simulink model "Sample594"  (R2021b)
settings: Solver=VariableStepAuto  StartTime=0.0  StopTime=10.0  RelTol=1e-3
undefined symbols (not defined in the file): DiscIntNeverNeededParam, magnitude, Newton, Raphson
libraries: simulink x402, pid_lib x98
(part 1 of 14)
settings Model: Creator=user  LastModifiedBy=汪海博

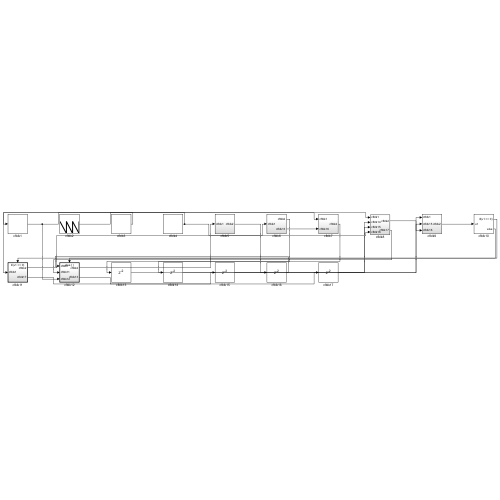
[thumbnail: Simulink's stored preview of the top-level diagram]
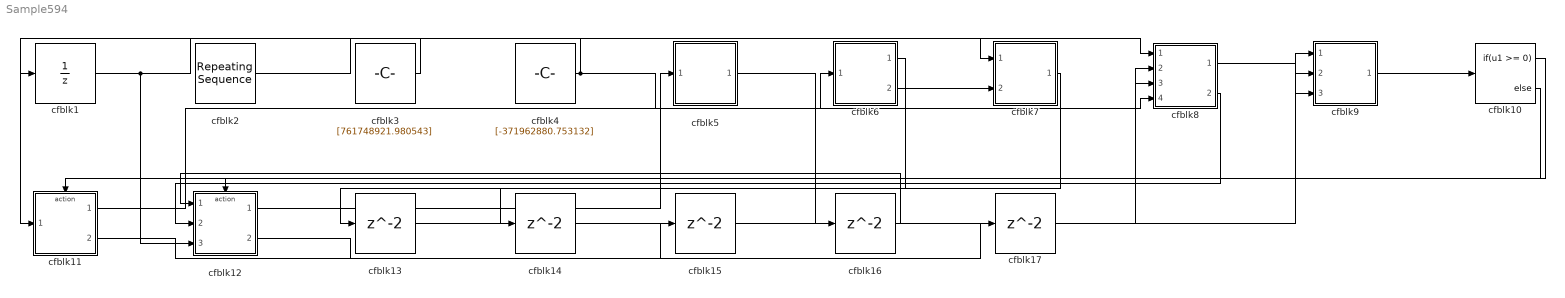
== system Sample594 ==
  cfblk1 : UnitDelay  HasFrameUpgradeWarning=on
  cfblk10 : If  IfExpression=u1 >= 0  SampleTime=1
  cfblk11 : Subsystem  TreatAsAtomicUnit=on
  cfblk12 : Subsystem  TreatAsAtomicUnit=on
  cfblk{13..17} (5 alike) : Delay  SampleTime=1
  cfblk2 : simulink/Sources/Repeating Sequence  rep_seq_t=[0 2]  rep_seq_y=[-284129757.481176, -754756546.872150]
  cfblk3 : Constant  Value=[761748921.980543]  SampleTime=1
  cfblk4 : Constant  Value=[-371962880.753132]  SampleTime=1
  cfblk5 : Subsystem
  cfblk6 : Subsystem
  cfblk7 : Subsystem
  cfblk8 : Subsystem
  cfblk9 : Subsystem
  wires:
  cfblk11/1(cfblk2) -> cfblk6/1(cfblk1)
  cfblk4/1 -> cfblk11/1(cfblk1), cfblk8/4(cfblk16)
  cfblk2/1 -> cfblk7/1(cfblk1)
  cfblk9/1(cfblk2) -> cfblk10/1
  cfblk3/1 -> cfblk1/1
  cfblk1/1 -> cfblk8/1(cfblk1), cfblk12/3(cfblk12)
  cfblk8/1(cfblk2) -> cfblk9/3(cfblk16)
  cfblk12/1(cfblk2) -> cfblk5/1(cfblk1)
  cfblk6/2(cfblk13) -> cfblk7/2(cfblk16)
  cfblk8/2(cfblk17) -> cfblk12/2(cfblk11)
  cfblk10/1 -> cfblk11/Action
  cfblk10/2 -> cfblk12/Action
  cfblk6/1(cfblk2) -> cfblk13/1
  cfblk13/1 -> cfblk9/2(cfblk15)
  cfblk7/1(cfblk2) -> cfblk14/1
  cfblk14/1 -> cfblk8/2(cfblk14)
  cfblk11/2(cfblk17) -> cfblk15/1
  cfblk15/1 -> cfblk9/1(cfblk1)
  cfblk5/1(cfblk2) -> cfblk16/1
  cfblk16/1 -> cfblk12/1(cfblk1)
  cfblk12/2(cfblk13) -> cfblk17/1
  cfblk17/1 -> cfblk8/3(cfblk15)

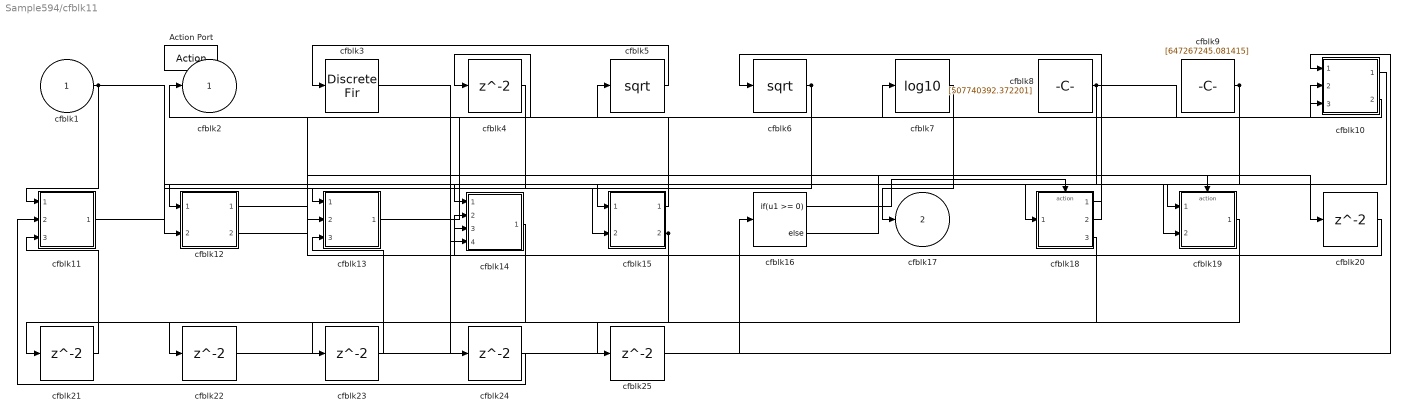
== system Sample594/cfblk11 ==
  cfblk1 : Inport
  Action Port : ActionPort  ActionPortLabel=if(u1 >= 0)
  cfblk10 : Subsystem
  cfblk11 : Subsystem
  cfblk12 : Subsystem
  cfblk13 : Subsystem
  cfblk14 : Subsystem
  cfblk15 : Subsystem
  cfblk16 : If  IfExpression=u1 >= 0  SampleTime=1
  cfblk18 : Subsystem  TreatAsAtomicUnit=on
  cfblk19 : Subsystem  TreatAsAtomicUnit=on
  cfblk{4,20..25} (7 alike) : Delay
  cfblk3 : DiscreteFir
  cfblk5 : Sqrt  SaturateOnIntegerOverflow=on
  cfblk6 : Sqrt  SaturateOnIntegerOverflow=on
  cfblk7 : Math  Operator=log10  SaturateOnIntegerOverflow=on
  cfblk8 : Constant  Value=[507740392.372201]  SampleTime=1
  cfblk9 : Constant  Value=[647267245.081415]  SampleTime=1
  cfblk2 : Outport
  cfblk17 : Outport  Port=2
  wires:
  cfblk1/1 -> cfblk11/1(cfblk1), cfblk19/2(cfblk8), cfblk15/2(cfblk9)
  cfblk8/1 -> cfblk12/1(cfblk1), cfblk10/3(cfblk15)
  cfblk11/1(cfblk2) -> cfblk13/1(cfblk1)
  cfblk18/1(cfblk2) -> cfblk6/1
  cfblk4/1 -> cfblk12/2(cfblk14)
  cfblk6/1 -> cfblk4/1, cfblk14/4(cfblk15)
  cfblk9/1 -> cfblk19/1(cfblk1), cfblk14/1(cfblk1)
  cfblk5/1 -> cfblk3/1
  cfblk12/2(cfblk15) -> cfblk7/1
  cfblk7/1 -> cfblk17/1
  cfblk18/2(cfblk12) -> cfblk15/1(cfblk1)
  cfblk15/1(cfblk2) -> cfblk2/1
  cfblk10/1(cfblk2) -> cfblk18/1(cfblk1)
  cfblk15/2(cfblk10) -> cfblk14/2(cfblk13), cfblk14/3(cfblk14), cfblk22/1
  cfblk13/1(cfblk2) -> cfblk10/2(cfblk14)
  cfblk10/2(cfblk16) -> cfblk5/1
  cfblk16/1 -> cfblk18/Action
  cfblk16/2 -> cfblk19/Action
  cfblk12/1(cfblk2) -> cfblk20/1
  cfblk20/1 -> cfblk13/2(cfblk10)
  cfblk14/1(cfblk2) -> cfblk21/1
  cfblk21/1 -> cfblk11/3(cfblk15)
  cfblk22/1 -> cfblk10/1(cfblk1)
  cfblk18/3(cfblk13) -> cfblk23/1
  cfblk23/1 -> cfblk13/3(cfblk11)
  cfblk3/1 -> cfblk24/1
  cfblk24/1 -> cfblk11/2(cfblk14)
  cfblk19/1(cfblk2) -> cfblk25/1
  cfblk25/1 -> cfblk16/1

== system Sample594/cfblk12 ==
  cfblk1 : Inport
  cfblk11 : Inport  Port=2
  cfblk12 : Inport  Port=3
  Action Port : ActionPort  ActionPortLabel=else
  cfblk10 : Subsystem
  cfblk14 : Delay
  cfblk3 : simulink/Discrete/Transfer Fcn Lead or Lag  PoleZ=0.95  ZeroZ=0.75  ICPrevOutput=0.0  ICPrevInput=0.0  DoSatur=off
      settings: SourceProductBaseCode=SL
  cfblk4 : Product  Inputs=*
  cfblk5 : Product  Inputs=**
  cfblk6 : Abs
  cfblk7 : Sum  Inputs=+-
  cfblk8 : Constant  Value=[-306003779.164927]  SampleTime=1
  cfblk9 : Subsystem
  cfblk2 : Outport
  cfblk13 : Outport  Port=2
  wires:
  cfblk6/1 -> cfblk9/1(cfblk1)
  cfblk11/1 -> cfblk7/1
  cfblk3/1 -> cfblk7/2, cfblk10/2(cfblk11)
  cfblk1/1 -> cfblk5/1
  cfblk8/1 -> cfblk4/1
  cfblk4/1 -> cfblk3/1
  cfblk10/1(cfblk2) -> cfblk13/1
  cfblk12/1 -> cfblk2/1
  cfblk7/1 -> cfblk5/2
  cfblk5/1 -> cfblk10/1(cfblk1)
  cfblk9/1(cfblk2) -> cfblk14/1
  cfblk14/1 -> cfblk6/1

== system Sample594/cfblk5 ==
  cfblk1 : Inport
  cfblk3 : simulink/Math Operations/MinMax Running Resettable  Function=min  vinit=0.0
  cfblk4 : Gain  Gain=[768236273.683915]
  cfblk5 : ComplexToMagnitudeAngle
  cfblk6 : Product  Inputs=**
  cfblk7 : Constant  Value=[-650989527.079987]  SampleTime=1
  cfblk8 : Subsystem
  cfblk9 : Delay  SampleTime=1
  cfblk2 : Outport
  wires:
  cfblk3/1 -> cfblk8/1(cfblk1)
  cfblk4/1 -> cfblk6/1
  cfblk7/1 -> cfblk8/2(cfblk9)
  cfblk8/1(cfblk2) -> cfblk4/1
  cfblk8/2(cfblk10) -> cfblk2/1
  cfblk1/1 -> cfblk5/1
  cfblk5/1 -> cfblk3/2
  cfblk5/2 -> cfblk6/2
  cfblk6/1 -> cfblk9/1
  cfblk9/1 -> cfblk3/1

== system Sample594/cfblk6 ==
  cfblk1 : Inport
  cfblk10 : Subsystem
  cfblk11 : Subsystem
  cfblk12 : Subsystem
  cfblk{3,14..18} (6 alike) : Delay  SampleTime=1
  cfblk4 : DiscreteFir  SampleTime=1
  cfblk5 : DotProduct  InputSameDT=on  OutDataTypeStr=Inherit: Inherit via internal rule
  cfblk6 : Math  Operator=hermitian  SaturateOnIntegerOverflow=on
  cfblk7 : Subsystem
  cfblk8 : Subsystem
  cfblk9 : Subsystem
  cfblk2 : Outport
  cfblk13 : Outport  Port=2
  wires:
  cfblk1/1 -> cfblk4/1
  cfblk10/1(cfblk2) -> cfblk9/1(cfblk1)
  cfblk4/1 -> cfblk11/1(cfblk1), cfblk12/2(cfblk11)
  cfblk10/2(cfblk10) -> cfblk3/1
  cfblk9/1(cfblk2) -> cfblk13/1
  cfblk5/1 -> cfblk8/1(cfblk1), cfblk10/2(cfblk9)
  cfblk8/1(cfblk2) -> cfblk7/1(cfblk1), cfblk15/1
  cfblk3/1 -> cfblk7/2(cfblk7)
  cfblk11/1(cfblk2) -> cfblk8/2(cfblk12)
  cfblk6/1 -> cfblk11/3(cfblk12), cfblk16/1
  cfblk12/1(cfblk2) -> cfblk2/1
  cfblk9/2(cfblk15) -> cfblk6/1
  cfblk10/3(cfblk11) -> cfblk9/2(cfblk14)
  cfblk10/4(cfblk12) -> cfblk12/1(cfblk1), cfblk18/1
  cfblk7/1(cfblk2) -> cfblk14/1
  cfblk14/1 -> cfblk11/2(cfblk11)
  cfblk15/1 -> cfblk11/4(cfblk13)
  cfblk16/1 -> cfblk5/1
  cfblk9/3(cfblk16) -> cfblk17/1
  cfblk17/1 -> cfblk10/1(cfblk1)
  cfblk18/1 -> cfblk5/2

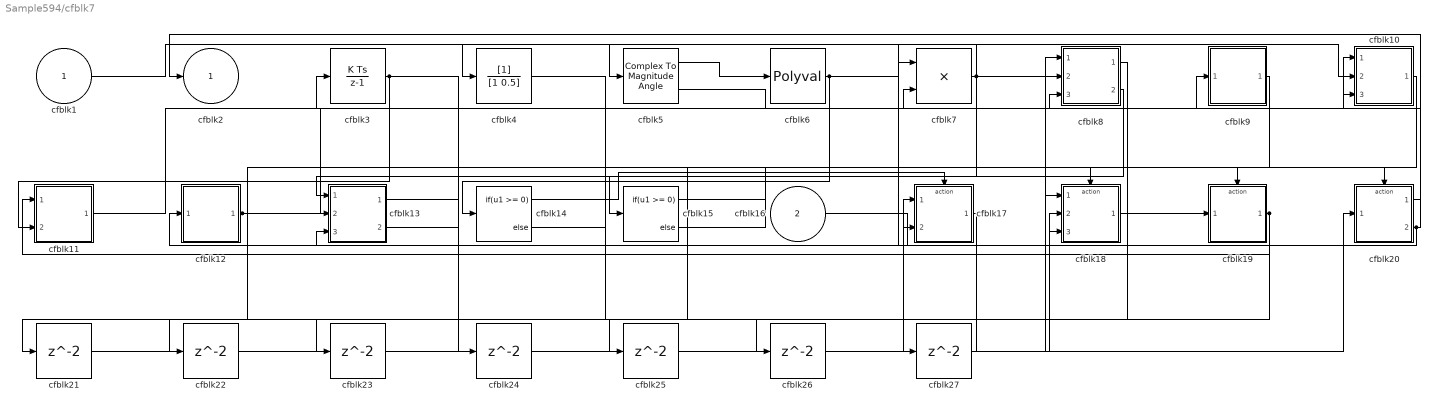
== system Sample594/cfblk7 ==
  cfblk1 : Inport
  cfblk16 : Inport  Port=2
  cfblk10 : Subsystem
  cfblk11 : Subsystem
  cfblk12 : Subsystem
  cfblk13 : Subsystem
  cfblk14 : If  IfExpression=u1 >= 0  SampleTime=1
  cfblk15 : If  IfExpression=u1 >= 0  SampleTime=1
  cfblk17 : Subsystem  TreatAsAtomicUnit=on
  cfblk18 : Subsystem  TreatAsAtomicUnit=on
  cfblk19 : Subsystem  TreatAsAtomicUnit=on
  cfblk20 : Subsystem  TreatAsAtomicUnit=on
  cfblk{21..27} (7 alike) : Delay  SampleTime=1
  cfblk3 : DiscreteIntegrator  ICPrevOutput=DiscIntNeverNeededParam  ICPrevScaledInput=DiscIntNeverNeededParam
  cfblk4 : DiscreteFilter  SampleTime=1
  cfblk5 : ComplexToMagnitudeAngle
  cfblk6 : Polyval  Coefs=[ +2.081618890e-019, -1.441693666e-014, +4.719686976e-010, -8.536869453e-006, +1.621573104e-001, -8.087801117e+001 ]
  cfblk7 : Product  Inputs=**
  cfblk8 : Subsystem
  cfblk9 : Subsystem
  cfblk2 : Outport
  wires:
  cfblk3/1 -> cfblk11/2(cfblk12), cfblk26/1
  cfblk5/1 -> cfblk6/1
  cfblk6/1 -> cfblk14/1, cfblk10/2(cfblk15)
  cfblk7/1 -> cfblk15/1, cfblk4/1, cfblk10/3(cfblk16)
  cfblk17/1(cfblk2) -> cfblk12/1(cfblk1)
  cfblk11/1(cfblk2) -> cfblk9/1(cfblk1)
  cfblk5/2 -> cfblk7/2
  cfblk16/1 -> cfblk18/2(cfblk11)
  cfblk20/1(cfblk2) -> cfblk2/1
  cfblk18/1(cfblk2) -> cfblk19/1(cfblk1)
  cfblk1/1 -> cfblk5/1
  cfblk20/2(cfblk7) -> cfblk3/1, cfblk17/1(cfblk1)
  cfblk13/2(cfblk16) -> cfblk10/1(cfblk1)
  cfblk12/1(cfblk2) -> cfblk8/3(cfblk16), cfblk13/2(cfblk14)
  cfblk19/1(cfblk2) -> cfblk11/1(cfblk1), cfblk13/3(cfblk15), cfblk23/1
  cfblk8/2(cfblk17) -> cfblk13/1(cfblk1)
  cfblk14/1 -> cfblk17/Action
  cfblk14/2 -> cfblk18/Action
  cfblk15/1 -> cfblk19/Action
  cfblk15/2 -> cfblk20/Action
  cfblk8/1(cfblk2) -> cfblk21/1
  cfblk21/1 -> cfblk18/3(cfblk12)
  cfblk9/1(cfblk2) -> cfblk22/1
  cfblk22/1 -> cfblk8/1(cfblk1)
  cfblk23/1 -> cfblk17/2(cfblk9)
  cfblk13/1(cfblk2) -> cfblk24/1
  cfblk24/1 -> cfblk18/1(cfblk1)
  cfblk10/1(cfblk2) -> cfblk25/1
  cfblk25/1 -> cfblk8/2(cfblk15)
  cfblk26/1 -> cfblk20/1(cfblk1)
  cfblk4/1 -> cfblk27/1
  cfblk27/1 -> cfblk7/1

== system Sample594/cfblk8 ==
  cfblk1 : Inport
  cfblk14 : Inport  Port=2
  cfblk15 : Inport  Port=3
  cfblk16 : Inport  Port=4
  cfblk10 : Subsystem
  cfblk11 : Subsystem
  cfblk12 : Subsystem
  cfblk13 : Subsystem
  cfblk{18..22} (5 alike) : Delay  SampleTime=1
  cfblk3 : DiscreteIntegrator  ICPrevOutput=DiscIntNeverNeededParam  ICPrevScaledInput=DiscIntNeverNeededParam
  cfblk4 : Delay  ShowEnablePort=on  SampleTime=1
      settings: InputPortMap=u0,e6
  cfblk5 : simulink/Math Operations/Slider Gain  gain=1  low=0  high=2
  cfblk6 : PermuteDimensions
  cfblk7 : Sqrt  SaturateOnIntegerOverflow=on
  cfblk8 : Constant  Value=[129507826.673968]  SampleTime=1
  cfblk9 : Subsystem
  cfblk2 : Outport
  cfblk17 : Outport  Port=2
  wires:
  cfblk16/1 -> cfblk10/1(cfblk1)
  cfblk6/1 -> cfblk17/1
  cfblk12/1(cfblk2) -> cfblk6/1
  cfblk3/1 -> cfblk9/1(cfblk1)
  cfblk7/1 -> cfblk11/1(cfblk1)
  cfblk13/1(cfblk2) -> cfblk4/1
  cfblk10/1(cfblk2) -> cfblk2/1
  cfblk11/1(cfblk2) -> cfblk5/1, cfblk20/1
  cfblk12/2(cfblk14) -> cfblk13/2(cfblk6)
  cfblk8/1 -> cfblk12/1(cfblk1)
  cfblk10/2(cfblk10) -> cfblk7/1
  cfblk10/3(cfblk11) -> cfblk21/1, cfblk22/1
  cfblk14/1 -> cfblk4/2
  cfblk9/1(cfblk2) -> cfblk10/2(cfblk9)
  cfblk5/1 -> cfblk12/2(cfblk13), cfblk19/1
  cfblk1/1 -> cfblk13/3(cfblk7)
  cfblk15/1 -> cfblk11/2(cfblk13)
  cfblk4/1 -> cfblk18/1
  cfblk18/1 -> cfblk13/1(cfblk1)
  cfblk19/1 -> cfblk11/3(cfblk14)
  cfblk20/1 -> cfblk9/3(cfblk12)
  cfblk21/1 -> cfblk3/1
  cfblk22/1 -> cfblk9/2(cfblk11)

== system Sample594/cfblk9 ==
  cfblk1 : Inport
  cfblk15 : Inport  Port=2
  cfblk16 : Inport  Port=3
  cfblk10 : Bias  Bias=[94307014.895825]
  cfblk11 : Assignment  DiagnosticForDimensions=Warning  IndexOptions=Index vector (dialog)  Indices=1  OutputSizes=1
  cfblk12 : Rounding
  cfblk13 : Constant  Value=[597719402.276021]  SampleTime=1
  cfblk14 : Subsystem
  cfblk{5,17..19} (4 alike) : Delay  SampleTime=1
  cfblk3 : simulink/Discrete/Transfer Fcn First Order  PoleZ=0.95  ICPrevOutput=0.0  DoSatur=off
  cfblk4 : DiscreteZeroPole  Poles=[0 0.5]  Gain=1
  cfblk6 : simulink/Discrete/Difference  ICPrevInput=0.0  OutMin=[]  OutMax=[]  OutDataTypeStr=Inherit: Inherit via back propagation  OutDataType=fixdt(1, 16)  OutScaling=2^-10  DoSatur=off
  cfblk7 : Trigonometry
  cfblk8 : Sum  Inputs=|++
  cfblk9 : ComplexToMagnitudeAngle
  cfblk2 : Outport
  wires:
  cfblk11/1 -> cfblk5/1
  cfblk5/1 -> cfblk10/1
  cfblk8/1 -> cfblk7/1
  cfblk15/1 -> cfblk3/1
  cfblk1/1 -> cfblk14/1(cfblk1)
  cfblk14/1(cfblk2) -> cfblk6/1
  cfblk3/1 -> cfblk9/1
  cfblk7/1 -> cfblk4/1
  cfblk14/2(cfblk14) -> cfblk12/1
  cfblk14/3(cfblk15) -> cfblk8/1
  cfblk14/4(cfblk16) -> cfblk2/1
  cfblk9/1 -> cfblk8/2
  cfblk13/1 -> cfblk14/3(cfblk11)
  cfblk12/1 -> cfblk11/1
  cfblk9/2 -> cfblk11/2
  cfblk6/1 -> cfblk17/1
  cfblk17/1 -> cfblk14/2(cfblk10)
  cfblk10/1 -> cfblk18/1
  cfblk18/1 -> cfblk14/4(cfblk12)
  cfblk4/1 -> cfblk19/1
  cfblk19/1 -> cfblk14/5(cfblk13)

== system Sample594/cfblk11/cfblk10 ==
  cfblk1 : Inport
  cfblk14 : Inport  Port=2
  cfblk15 : Inport  Port=3
  cfblk10 : Subsystem
  cfblk11 : Subsystem
  cfblk12 : Subsystem
  cfblk13 : Subsystem
  cfblk3 : simulink/Discrete/Difference  ICPrevInput=0.0  OutMin=[]  OutMax=[]  OutDataTypeStr=Inherit: Inherit via back propagation  OutDataType=fixdt(1, 16)  OutScaling=2^-10  DoSatur=off
  cfblk4 : pid_lib/PID Controller  Controller=PID  Form=Parallel  TimeDomain=Discrete-time  UseExternalTs=off  SampleTime=-1  IntegratorMethod=Forward Euler  FilterMethod=Forward Euler  ControllerParametersSource=internal  P=1  I=1  D=0  UseFilter=on  N=100  TunerSelectOption=Transfer Function Based (PID Tuner App)  InitialConditionSource=internal  InitialConditionForIntegrator=0  InitialConditionForFilter=0  DifferentiatorICPrevScaledInput=0  ExternalReset=none  TrackingMode=off  Kt=1  LimitOutput=off  SatLimitsSource=internal  UpperSaturationLimit=inf  LowerSaturationLimit=-inf  LinearizeAsGain=off  AntiWindupMode=none  Kb=1  POutMin=[]  POutMax=[]  IOutMin=[]  IOutMax=[]  DOutMin=[]  DOutMax=[]  NOutMin=[]  NOutMax=[]  SumOutMin=[]  SumOutMax=[]  SaturationOutMin=[]  SaturationOutMax=[]  PParamMin=[]  PParamMax=[]  IParamMin=[]  IParamMax=[]  DParamMin=[]  DParamMax=[]  NParamMin=[]  NParamMax=[]  KbParamMin=[]  KbParamMax=[]  KtParamMin=[]  KtParamMax=[]  KbOutMin=[]  KbOutMax=[]  KtOutMin=[]  KtOutMax=[]  IntegratorOutMin=[]  IntegratorOutMax=[]  FilterOutMin=[]  FilterOutMax=[]  SumI1OutMin=[]  SumI1OutMax=[]  SumI2OutMin=[]  SumI2OutMax=[]  SumI3OutMin=[]  SumI3OutMax=[]  SumI4OutMin=[]  SumI4OutMax=[]  SumDOutMin=[]  SumDOutMax=[]  DifferentiatorOutMin=[]  DifferentiatorOutMax=[]  FilterDiffOutCoefMin=[]  FilterDiffOutCoefMax=[]  ReciprocalOutMin=[]  ReciprocalOutMax=[]  SumDenOutMin=[]  SumDenOutMax=[]  SumNumOutMin=[]  SumNumOutMax=[]  DivideOutMin=[]  DivideOutMax=[]  UdiffTsProdOutMin=[]  UdiffTsProdOutMax=[]  NTsProdOutMin=[]  NTsProdOutMax=[]  UintegralTsProdOutMin=[]  UintegralTsProdOutMax=[]  UngainTsProdOutMin=[]  UngainTsProdOutMax=[]  IntegratorContinuousStateAttributes=''  IntegratorStateMustResolveToSignalObject=off  IntegratorRTWStateStorageClass=Auto  FilterContinuousStateAttributes=''  FilterStateMustResolveToSignalObject=off  FilterRTWStateStorageClass=Auto  ParallelPVariant=InternalParameters  IdealPVariant=Disabled  IVariant=InternalParameters  DVariant=InternalParameters  IntegratorVariant=Discrete  SatVariant=Disabled  AWVariant=Passthrough  PCopyVariant=Disabled  TRVariant=Disabled  FdbkBlocksVariant=Forward  IdealPFdbkVariant=Disabled  SatFdbkVariant=Disabled  DerivativeFilterVariant=ForwardEulerFilter  NVariant=InternalParameters  NCopyVariant=Disabled  FilterICVariant=InternalICsFilter  IntegratorICVariant=InternalICs  ExternalResetVariant=Disabled  TRSumVariant=Passthrough  SumFdbkVariant=Disabled  SumVariant=Sum_PID  TsampFilterVariant=InternalTs  TsampNgainVariant=Passthrough  TsampIntegralVariant=Passthrough  ExternalSaturationOutDataTypeStr=Inherit: Same as second input
  cfblk5 : Delay  DelayLengthSource=Input port
      settings: InputPortMap=u0,p1
  cfblk6 : simulink/Discrete/Transfer Fcn First Order  PoleZ=0.95  ICPrevOutput=0.0  DoSatur=off
  cfblk7 : Signum
  cfblk8 : Signum
  cfblk9 : Constant  Value=[55880807.632162]  SampleTime=1
  cfblk2 : Outport
  cfblk16 : Outport  Port=2
  wires:
  cfblk4/1 -> cfblk7/1
  cfblk8/1 -> cfblk11/1(cfblk1), cfblk13/2(cfblk12)
  cfblk11/1(cfblk2) -> cfblk3/1
  cfblk7/1 -> cfblk11/2(cfblk10)
  cfblk13/1(cfblk2) -> cfblk2/1
  cfblk6/1 -> cfblk8/1
  cfblk13/2(cfblk13) -> cfblk16/1
  cfblk12/1(cfblk2) -> cfblk13/1(cfblk1)
  cfblk15/1 -> cfblk10/1(cfblk1)
  cfblk3/1 -> cfblk5/1
  cfblk1/1 -> cfblk4/1
  cfblk14/1 -> cfblk5/2, cfblk6/1
  cfblk9/1 -> cfblk12/1(cfblk1)
  cfblk10/1(cfblk2) -> cfblk12/2(cfblk10)
  cfblk5/1 -> cfblk12/3(cfblk11)

== system Sample594/cfblk11/cfblk11 ==
  cfblk1 : Inport
  cfblk14 : Inport  Port=2
  cfblk15 : Inport  Port=3
  cfblk10 : Subsystem
  cfblk11 : Subsystem
  cfblk12 : Subsystem
  cfblk13 : If  IfExpression=u1 >= 0  SampleTime=1
  cfblk16 : Subsystem  TreatAsAtomicUnit=on
  cfblk17 : Subsystem  TreatAsAtomicUnit=on
  cfblk{18..22} (5 alike) : Delay
  cfblk3 : Delay  DelayLengthSource=Input port
      settings: InputPortMap=u0,p1
  cfblk4 : DiscreteZeroPole  Poles=[0 0.5]  Gain=1  SampleTime=-1
  cfblk5 : DiscreteZeroPole  Poles=[0 0.5]  Gain=1  SampleTime=-1
  cfblk6 : Sin  TimeSource=Use external signal  SampleTime=0
  cfblk7 : Rounding
  cfblk8 : Assignment  DiagnosticForDimensions=Warning  IndexOptions=Index vector (dialog)  Indices=1  OutputSizes=1
  cfblk9 : Product  Inputs=**
  cfblk2 : Outport
  wires:
  cfblk11/1(cfblk2) -> cfblk7/1
  cfblk14/1 -> cfblk5/1
  cfblk10/1(cfblk2) -> cfblk9/1
  cfblk5/1 -> cfblk16/1(cfblk1)
  cfblk7/1 -> cfblk18/1, cfblk20/1
  cfblk15/1 -> cfblk11/1(cfblk1)
  cfblk11/2(cfblk13) -> cfblk2/1
  cfblk12/1(cfblk2) -> cfblk11/2(cfblk10)
  cfblk9/1 -> cfblk4/1
  cfblk16/1(cfblk2) -> cfblk12/1(cfblk1)
  cfblk4/1 -> cfblk6/1
  cfblk3/1 -> cfblk13/1
  cfblk1/1 -> cfblk3/2, cfblk8/2, cfblk11/3(cfblk11)
  cfblk12/2(cfblk9) -> cfblk8/1
  cfblk12/3(cfblk10) -> cfblk10/1(cfblk1)
  cfblk12/4(cfblk11) -> cfblk10/2(cfblk9)
  cfblk13/1 -> cfblk16/Action
  cfblk13/2 -> cfblk17/Action
  cfblk18/1 -> cfblk17/1(cfblk1)
  cfblk17/1(cfblk2) -> cfblk19/1
  cfblk19/1 -> cfblk16/2(cfblk13)
  cfblk20/1 -> cfblk11/4(cfblk12)
  cfblk8/1 -> cfblk21/1
  cfblk21/1 -> cfblk3/1
  cfblk6/1 -> cfblk22/1
  cfblk22/1 -> cfblk9/2

== system Sample594/cfblk11/cfblk12 ==
  cfblk1 : Inport
  cfblk14 : Inport  Port=2
  cfblk10 : Constant  Value=[-282686673.263039]  SampleTime=1
  cfblk11 : Constant  Value=[-523176242.598219]  SampleTime=1
  cfblk12 : Subsystem
  cfblk13 : Subsystem
  cfblk16 : Delay
  cfblk17 : Delay
  cfblk3 : DiscreteFir
  cfblk4 : DiscreteFir
  cfblk5 : Trigonometry
  cfblk6 : Sum  Inputs=+-
  cfblk7 : Sum  Inputs=+-
  cfblk8 : Squeeze
  cfblk9 : DotProduct  InputSameDT=on  OutDataTypeStr=Inherit: Inherit via internal rule
  cfblk2 : Outport
  cfblk15 : Outport  Port=2
  wires:
  cfblk11/1 -> cfblk9/1
  cfblk6/1 -> cfblk13/1(cfblk1)
  cfblk10/1 -> cfblk8/1, cfblk7/2
  cfblk4/1 -> cfblk6/1
  cfblk13/1(cfblk2) -> cfblk5/1, cfblk17/1
  cfblk7/1 -> cfblk15/1
  cfblk3/1 -> cfblk2/1
  cfblk8/1 -> cfblk3/1
  cfblk9/1 -> cfblk7/1, cfblk12/3(cfblk13), cfblk13/2(cfblk7)
  cfblk12/1(cfblk2) -> cfblk4/1
  cfblk14/1 -> cfblk6/2
  cfblk1/1 -> cfblk12/2(cfblk12), cfblk9/2, cfblk13/3(cfblk8)
  cfblk5/1 -> cfblk16/1
  cfblk16/1 -> cfblk12/1(cfblk1)
  cfblk17/1 -> cfblk12/4(cfblk14)

== system Sample594/cfblk11/cfblk13 ==
  cfblk1 : Inport
  cfblk10 : Inport  Port=2
  cfblk11 : Inport  Port=3
  cfblk12 : Delay
  cfblk13 : Delay
  cfblk3 : Delay
  cfblk4 : Sum
  cfblk5 : Constant  Value=[-452128543.492404]  SampleTime=1
  cfblk6 : Constant  Value=[46654921.717771]  SampleTime=1
  cfblk7 : Subsystem
  cfblk8 : Subsystem
  cfblk9 : Subsystem
  cfblk2 : Outport
  wires:
  cfblk5/1 -> cfblk7/1(cfblk1)
  cfblk8/1(cfblk2) -> cfblk9/1(cfblk1)
  cfblk4/1 -> cfblk8/1(cfblk1)
  cfblk6/1 -> cfblk7/2(cfblk14)
  cfblk11/1 -> cfblk2/1
  cfblk9/1(cfblk2) -> cfblk7/3(cfblk15)
  cfblk10/1 -> cfblk3/1
  cfblk3/1 -> cfblk4/2
  cfblk7/1(cfblk2) -> cfblk12/1
  cfblk12/1 -> cfblk4/1
  cfblk9/2(cfblk12) -> cfblk13/1
  cfblk13/1 -> cfblk8/2(cfblk9)

== system Sample594/cfblk11/cfblk14 ==
  cfblk1 : Inport
  cfblk13 : Inport  Port=2
  cfblk14 : Inport  Port=3
  cfblk15 : Inport  Port=4
  cfblk10 : Subsystem
  cfblk11 : Subsystem
  cfblk12 : Subsystem
  cfblk16 : Delay
  cfblk17 : Delay
  cfblk3 : DiscreteStateSpace  SampleTime=-1
  cfblk4 : PermuteDimensions
  cfblk5 : Math  Operator=rem  SaturateOnIntegerOverflow=on
  cfblk6 : Reshape
  cfblk7 : Rounding
  cfblk8 : PermuteDimensions
  cfblk9 : Squeeze
  cfblk2 : Outport
  wires:
  cfblk8/1 -> cfblk10/1(cfblk1)
  cfblk3/1 -> cfblk2/1
  cfblk14/1 -> cfblk3/1
  cfblk7/1 -> cfblk11/1(cfblk1)
  cfblk4/1 -> cfblk6/1
  cfblk10/1(cfblk2) -> cfblk9/1
  cfblk12/1(cfblk2) -> cfblk8/1
  cfblk1/1 -> cfblk12/1(cfblk1)
  cfblk10/2(cfblk16) -> cfblk5/1
  cfblk10/3(cfblk17) -> cfblk4/1
  cfblk15/1 -> cfblk5/2
  cfblk9/1 -> cfblk16/1
  cfblk16/1 -> cfblk10/2(cfblk15)
  cfblk11/1(cfblk2) -> cfblk17/1
  cfblk17/1 -> cfblk7/1

== system Sample594/cfblk11/cfblk15 ==
  cfblk1 : Inport
  cfblk9 : Inport  Port=2
  cfblk3 : DiscreteFilter
  cfblk4 : simulink/Discrete/Transfer Fcn Real Zero  ZeroZ=0.75  ICPrevInput=0.0  DoSatur=off
      settings: SourceProductBaseCode=SL
  cfblk5 : PermuteDimensions
  cfblk6 : Constant  Value=[-953763112.290072]  SampleTime=1
  cfblk7 : Subsystem
  cfblk8 : Subsystem
  cfblk2 : Outport
  cfblk10 : Outport  Port=2
  wires:
  cfblk3/1 -> cfblk4/1
  cfblk1/1 -> cfblk7/1(cfblk1)
  cfblk4/1 -> cfblk7/2(cfblk8)
  cfblk6/1 -> cfblk8/1(cfblk1), cfblk3/1
  cfblk8/1(cfblk2) -> cfblk10/1, cfblk5/1
  cfblk5/1 -> cfblk2/1
  cfblk9/1 -> cfblk8/2(cfblk11)
  cfblk7/1(cfblk2) -> cfblk8/3(cfblk12)

== system Sample594/cfblk11/cfblk18 ==
  cfblk1 : Inport
  Action Port : ActionPort  ActionPortLabel=if(u1 >= 0)
  cfblk10 : Subsystem
  cfblk11 : Subsystem
  cfblk14 : Delay
  cfblk15 : Delay
  cfblk3 : simulink/Discrete/Transfer Fcn First Order  PoleZ=0.95  ICPrevOutput=0.0  DoSatur=off
  cfblk4 : DotProduct  InputSameDT=on  OutDataTypeStr=Inherit: Inherit via internal rule
  cfblk5 : UnaryMinus
  cfblk6 : Rounding
  cfblk7 : Bias  Bias=[167199444.959874]
  cfblk8 : Constant  Value=[837444211.495958]  SampleTime=1
  cfblk9 : Subsystem
  cfblk2 : Outport
  cfblk12 : Outport  Port=2
  cfblk13 : Outport  Port=3
  wires:
  cfblk5/1 -> cfblk13/1, cfblk14/1
  cfblk4/1 -> cfblk7/1, cfblk11/2(cfblk12), cfblk9/3(cfblk13)
  cfblk10/1(cfblk2) -> cfblk5/1
  cfblk1/1 -> cfblk6/1, cfblk9/4(cfblk14)
  cfblk11/1(cfblk2) -> cfblk10/2(cfblk13)
  cfblk9/1(cfblk2) -> cfblk12/1
  cfblk6/1 -> cfblk11/1(cfblk1), cfblk9/1(cfblk1), cfblk9/2(cfblk12)
  cfblk8/1 -> cfblk2/1, cfblk11/3(cfblk13), cfblk3/1
  cfblk3/1 -> cfblk4/2
  cfblk14/1 -> cfblk10/1(cfblk1)
  cfblk7/1 -> cfblk15/1
  cfblk15/1 -> cfblk4/1

== system Sample594/cfblk11/cfblk19 ==
  cfblk1 : Inport
  cfblk8 : Inport  Port=2
  Action Port : ActionPort  ActionPortLabel=else
  cfblk3 : Delay  DelayLengthSource=Input port
      settings: InputPortMap=u0,p1
  cfblk4 : MinMax  Function=max  Inputs=3
  cfblk5 : Constant  Value=[698763643.192819]  SampleTime=1
  cfblk6 : Subsystem
  cfblk7 : Subsystem
  cfblk2 : Outport
  wires:
  cfblk7/1(cfblk2) -> cfblk3/1
  cfblk3/1 -> cfblk6/1(cfblk1)
  cfblk8/1 -> cfblk7/1(cfblk1)
  cfblk1/1 -> cfblk3/2
  cfblk5/1 -> cfblk6/2(cfblk11)
  cfblk4/1 -> cfblk2/1
  cfblk6/1(cfblk2) -> cfblk4/1
  cfblk6/2(cfblk12) -> cfblk4/2
  cfblk6/3(cfblk13) -> cfblk4/3

== system Sample594/cfblk12/cfblk10 ==
  cfblk1 : Inport
  cfblk11 : Inport  Port=2
  cfblk10 : Subsystem
  cfblk13 : Delay
  cfblk3 : simulink/Discrete/Transfer Fcn Lead or Lag  PoleZ=0.95  ZeroZ=0.75  ICPrevOutput=0.0  ICPrevInput=0.0  DoSatur=off
      settings: SourceProductBaseCode=SL
  cfblk4 : pid_lib/PID Controller (2DOF)  Controller=PID  Form=Parallel  TimeDomain=Discrete-time  UseExternalTs=off  SampleTime=-1  IntegratorMethod=Forward Euler  FilterMethod=Forward Euler  ControllerParametersSource=internal  P=1  I=1  D=0  UseFilter=on  N=100  b=1  c=1  TunerSelectOption=Transfer Function Based (PID Tuner App)  InitialConditionSource=internal  InitialConditionForIntegrator=0  InitialConditionForFilter=0  DifferentiatorICPrevScaledInput=0  ExternalReset=none  TrackingMode=off  Kt=1  LimitOutput=off  SatLimitsSource=internal  UpperSaturationLimit=inf  LowerSaturationLimit=-inf  LinearizeAsGain=off  AntiWindupMode=none  Kb=1  POutMin=[]  POutMax=[]  IOutMin=[]  IOutMax=[]  DOutMin=[]  DOutMax=[]  NOutMin=[]  NOutMax=[]  bOutMin=[]  bOutMax=[]  cOutMin=[]  cOutMax=[]  SumOutMin=[]  SumOutMax=[]  SaturationOutMin=[]  SaturationOutMax=[]  PParamMin=[]  PParamMax=[]  IParamMin=[]  IParamMax=[]  DParamMin=[]  DParamMax=[]  NParamMin=[]  NParamMax=[]  bParamMin=[]  bParamMax=[]  cParamMin=[]  cParamMax=[]  KbParamMin=[]  KbParamMax=[]  KtParamMin=[]  KtParamMax=[]  KbOutMin=[]  KbOutMax=[]  KtOutMin=[]  KtOutMax=[]  IntegratorOutMin=[]  IntegratorOutMax=[]  FilterOutMin=[]  FilterOutMax=[]  SumI1OutMin=[]  SumI1OutMax=[]  SumI2OutMin=[]  SumI2OutMax=[]  SumI3OutMin=[]  SumI3OutMax=[]  SumI4OutMin=[]  SumI4OutMax=[]  SumDOutMin=[]  SumDOutMax=[]  Sum1OutMin=[]  Sum1OutMax=[]  Sum2OutMin=[]  Sum2OutMax=[]  Sum3OutMin=[]  Sum3OutMax=[]  DifferentiatorOutMin=[]  DifferentiatorOutMax=[]  FilterDiffOutCoefMin=[]  FilterDiffOutCoefMax=[]  ReciprocalOutMin=[]  ReciprocalOutMax=[]  SumDenOutMin=[]  SumDenOutMax=[]  SumNumOutMin=[]  SumNumOutMax=[]  DivideOutMin=[]  DivideOutMax=[]  UdiffTsProdOutMin=[]  UdiffTsProdOutMax=[]  NTsProdOutMin=[]  NTsProdOutMax=[]  UintegralTsProdOutMin=[]  UintegralTsProdOutMax=[]  UngainTsProdOutMin=[]  UngainTsProdOutMax=[]  IntegratorContinuousStateAttributes=''  IntegratorStateMustResolveToSignalObject=off  IntegratorRTWStateStorageClass=Auto  FilterContinuousStateAttributes=''  FilterStateMustResolveToSignalObject=off  FilterRTWStateStorageClass=Auto  ParallelPVariant=InternalParameters  IdealPVariant=Disabled  IVariant=InternalParameters  DVariant=InternalParameters  bVariant=InternalParameters  cVariant=InternalParameters  IntegratorVariant=Discrete  SatVariant=Disabled  AWVariant=Passthrough  PCopyVariant=Disabled  TRVariant=Disabled  FdbkBlocksVariant=Forward  IdealPFdbkVariant=Disabled  SatFdbkVariant=Disabled  DerivativeFilterVariant=ForwardEulerFilter  NVariant=InternalParameters  NCopyVariant=Disabled  FilterICVariant=InternalICsFilter  IntegratorICVariant=InternalICs  ExternalResetVariant=Disabled  TRSumVariant=Passthrough  SumFdbkVariant=Disabled  SumVariant=Sum_PID  TsampFilterVariant=InternalTs  TsampNgainVariant=Passthrough  TsampIntegralVariant=Passthrough  ExternalSaturationOutDataTypeStr=Inherit: Same as second input
      settings: SourceProductBaseCode=SL
  cfblk5 : simulink/Discrete/Tapped Delay  vinit=0.0  samptime=-1  NumDelays=1  DelayOrder=Oldest  includeCurrent=off
  cfblk6 : ComplexToMagnitudeAngle
  cfblk7 : Abs
  cfblk8 : Constant  Value=[406225975.976458]  SampleTime=1
  cfblk9 : Subsystem
  cfblk2 : Outport
  cfblk12 : Outport  Port=2
  wires:
  cfblk6/1 -> cfblk9/1(cfblk1)
  cfblk11/1 -> cfblk9/2(cfblk10)
  cfblk6/2 -> cfblk7/1
  cfblk4/1 -> cfblk3/1
  cfblk7/1 -> cfblk2/1
  cfblk5/1 -> cfblk10/1(cfblk1), cfblk10/3(cfblk11)
  cfblk9/1(cfblk2) -> cfblk12/1
  cfblk1/1 -> cfblk10/2(cfblk10)
  cfblk8/1 -> cfblk5/1
  cfblk10/1(cfblk2) -> cfblk4/1, cfblk6/1
  cfblk3/1 -> cfblk13/1
  cfblk13/1 -> cfblk4/2

== system Sample594/cfblk12/cfblk9 ==
  cfblk1 : Inport
  cfblk3 : DiscreteZeroPole  Poles=[0 0.5]  Gain=1  SampleTime=-1
  cfblk4 : Sum  Inputs=+
  cfblk5 : Subsystem
  cfblk6 : Subsystem
  cfblk7 : Subsystem
  cfblk8 : Delay
  cfblk9 : Delay
  cfblk2 : Outport
  wires:
  cfblk6/1(cfblk2) -> cfblk7/1(cfblk1)
  cfblk4/1 -> cfblk2/1
  cfblk5/1(cfblk2) -> cfblk4/1
  cfblk1/1 -> cfblk5/2(cfblk13)
  cfblk5/2(cfblk14) -> cfblk6/1(cfblk1)
  cfblk7/1(cfblk2) -> cfblk3/1, cfblk9/1
  cfblk3/1 -> cfblk8/1
  cfblk8/1 -> cfblk5/1(cfblk1)
  cfblk9/1 -> cfblk6/2(cfblk9)

== system Sample594/cfblk5/cfblk8 ==
  cfblk1 : Inport
  cfblk9 : Inport  Port=2
  cfblk11 : Delay  SampleTime=1
  cfblk3 : DiscreteFir  SampleTime=1
  cfblk4 : Squeeze
  cfblk5 : Sqrt  Operator=rSqrt  AlgorithmType=Newton-Raphson  SaturateOnIntegerOverflow=on
  cfblk6 : DotProduct  InputSameDT=on  OutDataTypeStr=Inherit: Inherit via internal rule
  cfblk7 : Subsystem
  cfblk8 : Subsystem
  cfblk2 : Outport
  cfblk10 : Outport  Port=2
  wires:
  cfblk3/1 -> cfblk10/1
  cfblk1/1 -> cfblk6/1, cfblk7/1(cfblk1)
  cfblk6/1 -> cfblk8/1(cfblk1)
  cfblk9/1 -> cfblk5/1
  cfblk7/1(cfblk2) -> cfblk4/1
  cfblk5/1 -> cfblk2/1
  cfblk7/2(cfblk15) -> cfblk8/2(cfblk12)
  cfblk4/1 -> cfblk3/1
  cfblk8/1(cfblk2) -> cfblk11/1
  cfblk11/1 -> cfblk6/2

== system Sample594/cfblk6/cfblk10 ==
  cfblk1 : Inport
  cfblk9 : Inport  Port=2
  cfblk3 : Product  Inputs=*
  cfblk4 : Squeeze
  cfblk5 : Signum
  cfblk6 : Subsystem
  cfblk7 : Subsystem
  cfblk8 : Subsystem
  cfblk2 : Outport
  cfblk10 : Outport  Port=2
  cfblk11 : Outport  Port=3
  cfblk12 : Outport  Port=4
  wires:
  cfblk7/1(cfblk2) -> cfblk2/1
  cfblk5/1 -> cfblk10/1
  cfblk7/2(cfblk12) -> cfblk6/1(cfblk1), cfblk6/3(cfblk13)
  cfblk6/1(cfblk2) -> cfblk5/1
  cfblk9/1 -> cfblk8/1(cfblk1)
  cfblk4/1 -> cfblk3/1, cfblk7/1(cfblk1), cfblk7/2(cfblk10)
  cfblk1/1 -> cfblk8/2(cfblk11), cfblk7/3(cfblk11), cfblk6/4(cfblk14), cfblk6/5(cfblk15)
  cfblk3/1 -> cfblk12/1
  cfblk8/1(cfblk2) -> cfblk4/1, cfblk6/2(cfblk12), cfblk11/1

== system Sample594/cfblk6/cfblk11 ==
  cfblk1 : Inport
  cfblk11 : Inport  Port=2
  cfblk12 : Inport  Port=3
  cfblk13 : Inport  Port=4
  cfblk10 : Subsystem
  cfblk3 : simulink/Discrete/Transfer Fcn First Order  PoleZ=0.95  ICPrevOutput=0.0  DoSatur=off
  cfblk4 : UnaryMinus
  cfblk5 : Sum  Inputs=|++
  cfblk6 : ComplexToMagnitudeAngle
  cfblk7 : Constant  Value=[-611654968.106405]  SampleTime=1
  cfblk8 : Constant  Value=[197960814.416167]  SampleTime=1
  cfblk9 : Subsystem
  cfblk2 : Outport
  wires:
  cfblk8/1 -> cfblk2/1
  cfblk1/1 -> cfblk5/1
  cfblk6/1 -> cfblk3/1
  cfblk10/1(cfblk2) -> cfblk4/1
  cfblk11/1 -> cfblk5/2
  cfblk3/1 -> cfblk9/1(cfblk1)
  cfblk7/1 -> cfblk6/1
  cfblk12/1 -> cfblk10/1(cfblk1)
  cfblk6/2 -> cfblk10/2(cfblk8)
  cfblk5/1 -> cfblk9/2(cfblk7)

== system Sample594/cfblk6/cfblk12 ==
  cfblk1 : Inport
  cfblk11 : Inport  Port=2
  cfblk10 : Subsystem
  cfblk3 : simulink/Discrete/Tapped Delay  vinit=0.0  samptime=-1  NumDelays=1  DelayOrder=Oldest  includeCurrent=off
  cfblk4 : Delay  DelayLengthSource=Input port  SampleTime=1
      settings: InputPortMap=u0,p1
  cfblk5 : Product
  cfblk6 : Abs
  cfblk7 : Sum  Inputs=-+
  cfblk8 : Constant  Value=[826680057.544718]  SampleTime=1
  cfblk9 : Subsystem
  cfblk2 : Outport
  wires:
  cfblk6/1 -> cfblk3/1, cfblk10/2(cfblk11)
  cfblk4/1 -> cfblk9/1(cfblk1)
  cfblk10/1(cfblk2) -> cfblk4/1
  cfblk7/1 -> cfblk2/1
  cfblk1/1 -> cfblk7/1
  cfblk11/1 -> cfblk6/1, cfblk5/2
  cfblk3/1 -> cfblk4/2
  cfblk9/1(cfblk2) -> cfblk5/1
  cfblk5/1 -> cfblk7/2
  cfblk8/1 -> cfblk10/1(cfblk1)

== system Sample594/cfblk6/cfblk7 ==
  cfblk1 : Inport
  cfblk7 : Inport  Port=2
  cfblk3 : Delay  DelayLengthSource=Input port  SampleTime=1
      settings: InputPortMap=u0,p1
  cfblk4 : Signum
  cfblk5 : Subsystem
  cfblk6 : Subsystem
  cfblk8 : Delay  SampleTime=1
  cfblk2 : Outport
  wires:
  cfblk7/1 -> cfblk4/1
  cfblk1/1 -> cfblk2/1
  cfblk4/1 -> cfblk5/1(cfblk1), cfblk6/3(cfblk13)
  cfblk5/1(cfblk2) -> cfblk3/2
  cfblk3/1 -> cfblk6/1(cfblk1)
  cfblk5/2(cfblk11) -> cfblk6/2(cfblk12)
  cfblk6/1(cfblk2) -> cfblk8/1
  cfblk8/1 -> cfblk3/1

== system Sample594/cfblk6/cfblk8 ==
  cfblk1 : Inport
  cfblk12 : Inport  Port=2
  cfblk10 : Subsystem
  cfblk11 : Subsystem
  cfblk13 : Delay  SampleTime=1
  cfblk14 : Delay  SampleTime=1
  cfblk3 : simulink/Discrete/Transfer Fcn First Order  PoleZ=0.95  ICPrevOutput=0.0  DoSatur=off
  cfblk4 : UnitDelay  HasFrameUpgradeWarning=on
  cfblk5 : Trigonometry
  cfblk6 : Abs
  cfblk7 : Sum  Inputs=+-
  cfblk8 : ComplexToRealImag
  cfblk9 : Sin  TimeSource=Use external signal  SampleTime=0
  cfblk2 : Outport
  wires:
  cfblk12/1 -> cfblk7/1
  cfblk10/1(cfblk2) -> cfblk11/1(cfblk1)
  cfblk11/1(cfblk2) -> cfblk2/1
  cfblk8/1 -> cfblk5/1
  cfblk1/1 -> cfblk9/1
  cfblk4/1 -> cfblk8/1
  cfblk7/1 -> cfblk11/2(cfblk8)
  cfblk8/2 -> cfblk10/1(cfblk1)
  cfblk3/1 -> cfblk6/1
  cfblk9/1 -> cfblk7/2
  cfblk5/1 -> cfblk11/3(cfblk9)
  cfblk6/1 -> cfblk13/1
  cfblk13/1 -> cfblk3/1
  cfblk10/2(cfblk9) -> cfblk14/1
  cfblk14/1 -> cfblk4/1

== system Sample594/cfblk6/cfblk9 ==
  cfblk1 : Inport
  cfblk14 : Inport  Port=2
  cfblk10 : Subsystem
  cfblk11 : Subsystem
  cfblk12 : Subsystem
  cfblk13 : Subsystem
  cfblk{17..22} (6 alike) : Delay  SampleTime=1
  cfblk3 : pid_lib/PID Controller  Controller=PID  Form=Parallel  TimeDomain=Discrete-time  UseExternalTs=off  SampleTime=1  IntegratorMethod=Forward Euler  FilterMethod=Forward Euler  ControllerParametersSource=internal  P=1  I=1  D=0  UseFilter=on  N=100  TunerSelectOption=Transfer Function Based (PID Tuner App)  InitialConditionSource=internal  InitialConditionForIntegrator=0  InitialConditionForFilter=0  DifferentiatorICPrevScaledInput=0  ExternalReset=none  TrackingMode=off  Kt=1  LimitOutput=off  SatLimitsSource=internal  UpperSaturationLimit=inf  LowerSaturationLimit=-inf  LinearizeAsGain=off  AntiWindupMode=none  Kb=1  POutMin=[]  POutMax=[]  IOutMin=[]  IOutMax=[]  DOutMin=[]  DOutMax=[]  NOutMin=[]  NOutMax=[]  SumOutMin=[]  SumOutMax=[]  SaturationOutMin=[]  SaturationOutMax=[]  PParamMin=[]  PParamMax=[]  IParamMin=[]  IParamMax=[]  DParamMin=[]  DParamMax=[]  NParamMin=[]  NParamMax=[]  KbParamMin=[]  KbParamMax=[]  KtParamMin=[]  KtParamMax=[]  KbOutMin=[]  KbOutMax=[]  KtOutMin=[]  KtOutMax=[]  IntegratorOutMin=[]  IntegratorOutMax=[]  FilterOutMin=[]  FilterOutMax=[]  SumI1OutMin=[]  SumI1OutMax=[]  SumI2OutMin=[]  SumI2OutMax=[]  SumI3OutMin=[]  SumI3OutMax=[]  SumI4OutMin=[]  SumI4OutMax=[]  SumDOutMin=[]  SumDOutMax=[]  DifferentiatorOutMin=[]  DifferentiatorOutMax=[]  FilterDiffOutCoefMin=[]  FilterDiffOutCoefMax=[]  ReciprocalOutMin=[]  ReciprocalOutMax=[]  SumDenOutMin=[]  SumDenOutMax=[]  SumNumOutMin=[]  SumNumOutMax=[]  DivideOutMin=[]  DivideOutMax=[]  UdiffTsProdOutMin=[]  UdiffTsProdOutMax=[]  NTsProdOutMin=[]  NTsProdOutMax=[]  UintegralTsProdOutMin=[]  UintegralTsProdOutMax=[]  UngainTsProdOutMin=[]  UngainTsProdOutMax=[]  IntegratorContinuousStateAttributes=''  IntegratorStateMustResolveToSignalObject=off  IntegratorRTWStateStorageClass=Auto  FilterContinuousStateAttributes=''  FilterStateMustResolveToSignalObject=off  FilterRTWStateStorageClass=Auto  ParallelPVariant=InternalParameters  IdealPVariant=Disabled  IVariant=InternalParameters  DVariant=InternalParameters  IntegratorVariant=Discrete  SatVariant=Disabled  AWVariant=Passthrough  PCopyVariant=Disabled  TRVariant=Disabled  FdbkBlocksVariant=Forward  IdealPFdbkVariant=Disabled  SatFdbkVariant=Disabled  DerivativeFilterVariant=ForwardEulerFilter  NVariant=InternalParameters  NCopyVariant=Disabled  FilterICVariant=InternalICsFilter  IntegratorICVariant=InternalICs  ExternalResetVariant=Disabled  TRSumVariant=Passthrough  SumFdbkVariant=Disabled  SumVariant=Sum_PID  TsampFilterVariant=InternalTs  TsampNgainVariant=Passthrough  TsampIntegralVariant=Passthrough  ExternalSaturationOutDataTypeStr=Inherit: Same as second input
  cfblk4 : simulink/Discrete/Difference  ICPrevInput=0.0  OutMin=[]  OutMax=[]  OutDataTypeStr=Inherit: Inherit via back propagation  OutDataType=fixdt(1, 16)  OutScaling=2^-10  DoSatur=off
  cfblk5 : Gain  Gain=[-945650307.001060]
  cfblk6 : Trigonometry
  cfblk7 : Gain  Gain=[874388778.651656]
  cfblk8 : Subsystem
  cfblk9 : Subsystem
  cfblk2 : Outport
  cfblk15 : Outport  Port=2
  cfblk16 : Outport  Port=3
  wires:
  cfblk6/1 -> cfblk4/1, cfblk9/2(cfblk7)
  cfblk13/1(cfblk2) -> cfblk15/1
  cfblk1/1 -> cfblk7/1
  cfblk8/1(cfblk2) -> cfblk11/1(cfblk1)
  cfblk8/2(cfblk13) -> cfblk13/1(cfblk1), cfblk22/1
  cfblk11/1(cfblk2) -> cfblk6/1
  cfblk9/1(cfblk2) -> cfblk3/1, cfblk20/1
  cfblk4/1 -> cfblk16/1, cfblk17/1, cfblk18/1
  cfblk7/1 -> cfblk12/1(cfblk1)
  cfblk14/1 -> cfblk12/3(cfblk8), cfblk8/3(cfblk12)
  cfblk10/1(cfblk2) -> cfblk8/1(cfblk1)
  cfblk5/1 -> cfblk8/2(cfblk11), cfblk9/3(cfblk8)
  cfblk12/1(cfblk2) -> cfblk10/3(cfblk14)
  cfblk10/2(cfblk15) -> cfblk5/1
  cfblk12/2(cfblk9) -> cfblk2/1
  cfblk17/1 -> cfblk10/2(cfblk13)
  cfblk18/1 -> cfblk11/2(cfblk8)
  cfblk3/1 -> cfblk19/1
  cfblk19/1 -> cfblk9/1(cfblk1)
  cfblk20/1 -> cfblk11/3(cfblk9)
  cfblk11/2(cfblk10) -> cfblk21/1
  cfblk21/1 -> cfblk12/2(cfblk7)
  cfblk22/1 -> cfblk10/1(cfblk1)

== system Sample594/cfblk7/cfblk10 ==
  cfblk1 : Inport
  cfblk15 : Inport  Port=2
  cfblk16 : Inport  Port=3
  cfblk10 : Subsystem
  cfblk11 : Subsystem
  cfblk12 : Subsystem
  cfblk13 : Subsystem
  cfblk14 : Subsystem
  cfblk17 : Delay  SampleTime=1
  cfblk18 : Delay  SampleTime=1
  cfblk3 : Delay  ShowEnablePort=on  SampleTime=1
      settings: InputPortMap=u0,e6
  cfblk4 : simulink/Math Operations/Slider Gain  gain=1  low=0  high=2
  cfblk5 : Math  Operator=pow  SaturateOnIntegerOverflow=on
  cfblk6 : DotProduct  InputSameDT=on  OutDataTypeStr=Inherit: Inherit via internal rule
  cfblk7 : Subsystem
  cfblk8 : Subsystem
  cfblk9 : Subsystem
  cfblk2 : Outport
  wires:
  cfblk3/1 -> cfblk6/1
  cfblk11/1(cfblk2) -> cfblk9/1(cfblk1)
  cfblk8/1(cfblk2) -> cfblk2/1
  cfblk5/1 -> cfblk7/1(cfblk1), cfblk11/2(cfblk8)
  cfblk15/1 -> cfblk10/2(cfblk12)
  cfblk16/1 -> cfblk14/1(cfblk1)
  cfblk9/1(cfblk2) -> cfblk7/2(cfblk16), cfblk3/2
  cfblk14/1(cfblk2) -> cfblk8/1(cfblk1)
  cfblk11/2(cfblk9) -> cfblk8/2(cfblk8)
  cfblk12/1(cfblk2) -> cfblk13/1(cfblk1)
  cfblk4/1 -> cfblk3/1, cfblk9/2(cfblk10)
  cfblk14/2(cfblk8) -> cfblk10/3(cfblk13), cfblk4/1
  cfblk10/1(cfblk2) -> cfblk13/2(cfblk7)
  cfblk7/1(cfblk2) -> cfblk8/3(cfblk9)
  cfblk1/1 -> cfblk5/2
  cfblk10/2(cfblk14) -> cfblk11/1(cfblk1)
  cfblk10/3(cfblk15) -> cfblk6/2
  cfblk10/4(cfblk16) -> cfblk13/3(cfblk8)
  cfblk10/5(cfblk17) -> cfblk12/1(cfblk1)
  cfblk6/1 -> cfblk17/1
  cfblk17/1 -> cfblk5/1
  cfblk13/1(cfblk2) -> cfblk18/1
  cfblk18/1 -> cfblk10/1(cfblk1)

== system Sample594/cfblk7/cfblk11 ==
  cfblk1 : Inport
  cfblk12 : Inport  Port=2
  cfblk10 : Subsystem
  cfblk11 : Subsystem
  cfblk13 : Delay  SampleTime=1
  cfblk14 : Delay  SampleTime=1
  cfblk15 : Delay  SampleTime=1
  cfblk3 : UnitDelay  HasFrameUpgradeWarning=on
  cfblk4 : UnitDelay  HasFrameUpgradeWarning=on
  cfblk5 : DiscreteFilter  SampleTime=1
  cfblk6 : Reshape
  cfblk7 : Sum
  cfblk8 : Gain  Gain=[-181423075.070824]
  cfblk9 : Subsystem
  cfblk2 : Outport
  wires:
  cfblk5/1 -> cfblk10/1(cfblk1)
  cfblk10/1(cfblk2) -> cfblk2/1
  cfblk6/1 -> cfblk7/2, cfblk15/1
  cfblk12/1 -> cfblk11/1(cfblk1)
  cfblk3/1 -> cfblk4/1
  cfblk4/1 -> cfblk9/2(cfblk9), cfblk9/4(cfblk11)
  cfblk8/1 -> cfblk6/1, cfblk10/3(cfblk7), cfblk14/1
  cfblk1/1 -> cfblk5/1
  cfblk11/1(cfblk2) -> cfblk8/1
  cfblk9/1(cfblk2) -> cfblk7/1
  cfblk9/2(cfblk12) -> cfblk11/2(cfblk9), cfblk10/2(cfblk6)
  cfblk7/1 -> cfblk13/1
  cfblk13/1 -> cfblk3/1
  cfblk14/1 -> cfblk9/3(cfblk10)
  cfblk15/1 -> cfblk9/1(cfblk1)

== system Sample594/cfblk7/cfblk12 ==
  cfblk1 : Inport
  cfblk{10..13} (4 alike) : Delay  SampleTime=1
  cfblk3 : ComplexToMagnitudeAngle
  cfblk4 : MinMax  Function=max  Inputs=2
  cfblk5 : Constant  Value=[426105487.631959]  SampleTime=1
  cfblk6 : Subsystem
  cfblk7 : Subsystem
  cfblk8 : Subsystem
  cfblk9 : Subsystem
  cfblk2 : Outport
  wires:
  cfblk7/1(cfblk2) -> cfblk3/1
  cfblk9/1(cfblk2) -> cfblk10/1, cfblk11/1
  cfblk1/1 -> cfblk4/1
  cfblk8/1(cfblk2) -> cfblk9/1(cfblk1), cfblk12/1
  cfblk6/1(cfblk2) -> cfblk2/1, cfblk7/1(cfblk1)
  cfblk3/1 -> cfblk8/2(cfblk8)
  cfblk5/1 -> cfblk9/2(cfblk10), cfblk6/3(cfblk15), cfblk6/4(cfblk16)
  cfblk4/1 -> cfblk6/2(cfblk14), cfblk7/3(cfblk16)
  cfblk10/1 -> cfblk8/1(cfblk1)
  cfblk11/1 -> cfblk4/2
  cfblk12/1 -> cfblk7/2(cfblk15)
  cfblk3/2 -> cfblk13/1
  cfblk13/1 -> cfblk6/1(cfblk1)

== system Sample594/cfblk7/cfblk13 ==
  cfblk1 : Inport
  cfblk14 : Inport  Port=2
  cfblk15 : Inport  Port=3
  cfblk10 : Constant  Value=[699155748.928442]  SampleTime=1
  cfblk11 : Subsystem
  cfblk12 : Subsystem
  cfblk13 : If  IfExpression=u1 >= 0  SampleTime=1
  cfblk17 : Subsystem  TreatAsAtomicUnit=on
  cfblk18 : Subsystem  TreatAsAtomicUnit=on
  cfblk19 : Delay  SampleTime=1
  cfblk3 : DiscreteTransferFcn  SampleTime=1
  cfblk4 : simulink/Discrete/Tapped Delay  vinit=0.0  samptime=-1  NumDelays=1  DelayOrder=Oldest  includeCurrent=off
  cfblk5 : simulink/Discrete/Transfer Fcn Lead or Lag  PoleZ=0.95  ZeroZ=0.75  ICPrevOutput=0.0  ICPrevInput=0.0  DoSatur=off
      settings: SourceProductBaseCode=SL
  cfblk6 : pid_lib/PID Controller  Controller=PID  Form=Parallel  TimeDomain=Discrete-time  UseExternalTs=off  SampleTime=1  IntegratorMethod=Forward Euler  FilterMethod=Forward Euler  ControllerParametersSource=internal  P=1  I=1  D=0  UseFilter=on  N=100  TunerSelectOption=Transfer Function Based (PID Tuner App)  InitialConditionSource=internal  InitialConditionForIntegrator=0  InitialConditionForFilter=0  DifferentiatorICPrevScaledInput=0  ExternalReset=none  TrackingMode=off  Kt=1  LimitOutput=off  SatLimitsSource=internal  UpperSaturationLimit=inf  LowerSaturationLimit=-inf  LinearizeAsGain=off  AntiWindupMode=none  Kb=1  POutMin=[]  POutMax=[]  IOutMin=[]  IOutMax=[]  DOutMin=[]  DOutMax=[]  NOutMin=[]  NOutMax=[]  SumOutMin=[]  SumOutMax=[]  SaturationOutMin=[]  SaturationOutMax=[]  PParamMin=[]  PParamMax=[]  IParamMin=[]  IParamMax=[]  DParamMin=[]  DParamMax=[]  NParamMin=[]  NParamMax=[]  KbParamMin=[]  KbParamMax=[]  KtParamMin=[]  KtParamMax=[]  KbOutMin=[]  KbOutMax=[]  KtOutMin=[]  KtOutMax=[]  IntegratorOutMin=[]  IntegratorOutMax=[]  FilterOutMin=[]  FilterOutMax=[]  SumI1OutMin=[]  SumI1OutMax=[]  SumI2OutMin=[]  SumI2OutMax=[]  SumI3OutMin=[]  SumI3OutMax=[]  SumI4OutMin=[]  SumI4OutMax=[]  SumDOutMin=[]  SumDOutMax=[]  DifferentiatorOutMin=[]  DifferentiatorOutMax=[]  FilterDiffOutCoefMin=[]  FilterDiffOutCoefMax=[]  ReciprocalOutMin=[]  ReciprocalOutMax=[]  SumDenOutMin=[]  SumDenOutMax=[]  SumNumOutMin=[]  SumNumOutMax=[]  DivideOutMin=[]  DivideOutMax=[]  UdiffTsProdOutMin=[]  UdiffTsProdOutMax=[]  NTsProdOutMin=[]  NTsProdOutMax=[]  UintegralTsProdOutMin=[]  UintegralTsProdOutMax=[]  UngainTsProdOutMin=[]  UngainTsProdOutMax=[]  IntegratorContinuousStateAttributes=''  IntegratorStateMustResolveToSignalObject=off  IntegratorRTWStateStorageClass=Auto  FilterContinuousStateAttributes=''  FilterStateMustResolveToSignalObject=off  FilterRTWStateStorageClass=Auto  ParallelPVariant=InternalParameters  IdealPVariant=Disabled  IVariant=InternalParameters  DVariant=InternalParameters  IntegratorVariant=Discrete  SatVariant=Disabled  AWVariant=Passthrough  PCopyVariant=Disabled  TRVariant=Disabled  FdbkBlocksVariant=Forward  IdealPFdbkVariant=Disabled  SatFdbkVariant=Disabled  DerivativeFilterVariant=ForwardEulerFilter  NVariant=InternalParameters  NCopyVariant=Disabled  FilterICVariant=InternalICsFilter  IntegratorICVariant=InternalICs  ExternalResetVariant=Disabled  TRSumVariant=Passthrough  SumFdbkVariant=Disabled  SumVariant=Sum_PID  TsampFilterVariant=InternalTs  TsampNgainVariant=Passthrough  TsampIntegralVariant=Passthrough  ExternalSaturationOutDataTypeStr=Inherit: Same as second input
  cfblk7 : Sqrt  SaturateOnIntegerOverflow=on
  cfblk8 : Reshape
  cfblk9 : Sum  Inputs=|++
  cfblk2 : Outport
  cfblk16 : Outport  Port=2
  wires:
  cfblk18/1(cfblk2) -> cfblk7/1
  cfblk3/1 -> cfblk12/1(cfblk1)
  cfblk7/1 -> cfblk8/1
  cfblk10/1 -> cfblk5/1
  cfblk9/1 -> cfblk16/1
  cfblk1/1 -> cfblk11/1(cfblk1)
  cfblk8/1 -> cfblk12/2(cfblk14)
  cfblk4/1 -> cfblk17/1(cfblk1)
  cfblk12/1(cfblk2) -> cfblk9/1
  cfblk12/2(cfblk15) -> cfblk6/1
  cfblk5/1 -> cfblk3/1
  cfblk14/1 -> cfblk9/2
  cfblk6/1 -> cfblk2/1
  cfblk11/1(cfblk2) -> cfblk18/1(cfblk1)
  cfblk15/1 -> cfblk13/1
  cfblk13/1 -> cfblk17/Action
  cfblk13/2 -> cfblk18/Action
  cfblk17/1(cfblk2) -> cfblk19/1
  cfblk19/1 -> cfblk4/1

== system Sample594/cfblk7/cfblk17 ==
  cfblk1 : Inport
  cfblk9 : Inport  Port=2
  Action Port : ActionPort  ActionPortLabel=if(u1 >= 0)
  cfblk10 : Delay
  cfblk3 : pid_lib/PID Controller (2DOF)  Controller=PID  Form=Parallel  TimeDomain=Discrete-time  UseExternalTs=off  SampleTime=-1  IntegratorMethod=Forward Euler  FilterMethod=Forward Euler  ControllerParametersSource=internal  P=1  I=1  D=0  UseFilter=on  N=100  b=1  c=1  TunerSelectOption=Transfer Function Based (PID Tuner App)  InitialConditionSource=internal  InitialConditionForIntegrator=0  InitialConditionForFilter=0  DifferentiatorICPrevScaledInput=0  ExternalReset=none  TrackingMode=off  Kt=1  LimitOutput=off  SatLimitsSource=internal  UpperSaturationLimit=inf  LowerSaturationLimit=-inf  LinearizeAsGain=off  AntiWindupMode=none  Kb=1  POutMin=[]  POutMax=[]  IOutMin=[]  IOutMax=[]  DOutMin=[]  DOutMax=[]  NOutMin=[]  NOutMax=[]  bOutMin=[]  bOutMax=[]  cOutMin=[]  cOutMax=[]  SumOutMin=[]  SumOutMax=[]  SaturationOutMin=[]  SaturationOutMax=[]  PParamMin=[]  PParamMax=[]  IParamMin=[]  IParamMax=[]  DParamMin=[]  DParamMax=[]  NParamMin=[]  NParamMax=[]  bParamMin=[]  bParamMax=[]  cParamMin=[]  cParamMax=[]  KbParamMin=[]  KbParamMax=[]  KtParamMin=[]  KtParamMax=[]  KbOutMin=[]  KbOutMax=[]  KtOutMin=[]  KtOutMax=[]  IntegratorOutMin=[]  IntegratorOutMax=[]  FilterOutMin=[]  FilterOutMax=[]  SumI1OutMin=[]  SumI1OutMax=[]  SumI2OutMin=[]  SumI2OutMax=[]  SumI3OutMin=[]  SumI3OutMax=[]  SumI4OutMin=[]  SumI4OutMax=[]  SumDOutMin=[]  SumDOutMax=[]  Sum1OutMin=[]  Sum1OutMax=[]  Sum2OutMin=[]  Sum2OutMax=[]  Sum3OutMin=[]  Sum3OutMax=[]  DifferentiatorOutMin=[]  DifferentiatorOutMax=[]  FilterDiffOutCoefMin=[]  FilterDiffOutCoefMax=[]  ReciprocalOutMin=[]  ReciprocalOutMax=[]  SumDenOutMin=[]  SumDenOutMax=[]  SumNumOutMin=[]  SumNumOutMax=[]  DivideOutMin=[]  DivideOutMax=[]  UdiffTsProdOutMin=[]  UdiffTsProdOutMax=[]  NTsProdOutMin=[]  NTsProdOutMax=[]  UintegralTsProdOutMin=[]  UintegralTsProdOutMax=[]  UngainTsProdOutMin=[]  UngainTsProdOutMax=[]  IntegratorContinuousStateAttributes=''  IntegratorStateMustResolveToSignalObject=off  IntegratorRTWStateStorageClass=Auto  FilterContinuousStateAttributes=''  FilterStateMustResolveToSignalObject=off  FilterRTWStateStorageClass=Auto  ParallelPVariant=InternalParameters  IdealPVariant=Disabled  IVariant=InternalParameters  DVariant=InternalParameters  bVariant=InternalParameters  cVariant=InternalParameters  IntegratorVariant=Discrete  SatVariant=Disabled  AWVariant=Passthrough  PCopyVariant=Disabled  TRVariant=Disabled  FdbkBlocksVariant=Forward  IdealPFdbkVariant=Disabled  SatFdbkVariant=Disabled  DerivativeFilterVariant=ForwardEulerFilter  NVariant=InternalParameters  NCopyVariant=Disabled  FilterICVariant=InternalICsFilter  IntegratorICVariant=InternalICs  ExternalResetVariant=Disabled  TRSumVariant=Passthrough  SumFdbkVariant=Disabled  SumVariant=Sum_PID  TsampFilterVariant=InternalTs  TsampNgainVariant=Passthrough  TsampIntegralVariant=Passthrough  ExternalSaturationOutDataTypeStr=Inherit: Same as second input
      settings: SourceProductBaseCode=SL
  cfblk4 : DiscreteIntegrator  SampleTime=-1  ICPrevOutput=DiscIntNeverNeededParam  ICPrevScaledInput=DiscIntNeverNeededParam
  cfblk5 : simulink/Math Operations/Slider Gain  gain=1  low=0  high=2
  cfblk6 : Constant  Value=[-750166590.988642]  SampleTime=1
  cfblk7 : Constant  Value=[119572025.475577]  SampleTime=1
  cfblk8 : Subsystem
  cfblk2 : Outport
  wires:
  cfblk4/1 -> cfblk8/1(cfblk1)
  cfblk6/1 -> cfblk2/1
  cfblk3/1 -> cfblk5/1
  cfblk7/1 -> cfblk3/1
  cfblk1/1 -> cfblk3/2
  cfblk8/1(cfblk2) -> cfblk10/1
  cfblk10/1 -> cfblk4/1

== system Sample594/cfblk7/cfblk18 ==
  cfblk1 : Inport
  cfblk11 : Inport  Port=2
  cfblk12 : Inport  Port=3
  Action Port : ActionPort  ActionPortLabel=else
  cfblk10 : Subsystem
  cfblk13 : Delay
  cfblk14 : Delay
  cfblk3 : ComplexToRealImag
  cfblk4 : Product
  cfblk5 : Sum  Inputs=|++
  cfblk6 : Rounding
  cfblk7 : Product
  cfblk8 : Rounding
  cfblk9 : Subsystem
  cfblk2 : Outport
  wires:
  cfblk10/1(cfblk2) -> cfblk4/1
  cfblk8/1 -> cfblk2/1
  cfblk11/1 -> cfblk8/1
  cfblk3/1 -> cfblk7/1
  cfblk5/1 -> cfblk6/1
  cfblk12/1 -> cfblk7/2
  cfblk7/1 -> cfblk10/2(cfblk14), cfblk5/1
  cfblk3/2 -> cfblk4/2, cfblk5/2
  cfblk1/1 -> cfblk9/1(cfblk1)
  cfblk9/1(cfblk2) -> cfblk10/3(cfblk15)
  cfblk4/1 -> cfblk13/1
  cfblk13/1 -> cfblk10/1(cfblk1)
  cfblk6/1 -> cfblk14/1
  cfblk14/1 -> cfblk3/1

== system Sample594/cfblk7/cfblk19 ==
  cfblk1 : Inport
  Action Port : ActionPort  ActionPortLabel=if(u1 >= 0)
  cfblk3 : DiscreteFilter
  cfblk4 : simulink/Discrete/Transfer Fcn Real Zero  ZeroZ=0.75  ICPrevInput=0.0  DoSatur=off
      settings: SourceProductBaseCode=SL
  cfblk5 : Bias  Bias=[-278652910.278158]
  cfblk6 : Constant  Value=[767506550.536831]  SampleTime=1
  cfblk7 : Subsystem
  cfblk8 : Delay
  cfblk2 : Outport
  wires:
  cfblk4/1 -> cfblk5/1
  cfblk3/1 -> cfblk2/1
  cfblk5/1 -> cfblk3/1, cfblk8/1
  cfblk1/1 -> cfblk7/1(cfblk1)
  cfblk7/1(cfblk2) -> cfblk4/1
  cfblk6/1 -> cfblk7/2(cfblk11)
  cfblk8/1 -> cfblk7/3(cfblk12)

== system Sample594/cfblk7/cfblk20 ==
  cfblk1 : Inport
  Action Port : ActionPort  ActionPortLabel=else
  cfblk{8..11} (4 alike) : Delay
  cfblk3 : Delay  DelayLengthSource=Input port
      settings: InputPortMap=u0,p1
  cfblk4 : simulink/Math Operations/Slider Gain  gain=1  low=0  high=2
  cfblk5 : Subsystem
  cfblk6 : Subsystem
  cfblk2 : Outport
  cfblk7 : Outport  Port=2
  wires:
  cfblk4/1 -> cfblk7/1, cfblk5/2(cfblk16), cfblk5/3(cfblk17)
  cfblk5/1(cfblk2) -> cfblk3/1, cfblk9/1, cfblk10/1, cfblk11/1
  cfblk1/1 -> cfblk2/1, cfblk6/5(cfblk9)
  cfblk6/1(cfblk2) -> cfblk4/1
  cfblk6/2(cfblk10) -> cfblk5/1(cfblk1), cfblk3/2
  cfblk3/1 -> cfblk8/1
  cfblk8/1 -> cfblk6/1(cfblk1)
  cfblk9/1 -> cfblk6/2(cfblk6)
  cfblk10/1 -> cfblk6/3(cfblk7)
  cfblk11/1 -> cfblk6/4(cfblk8)

== system Sample594/cfblk7/cfblk8 ==
  cfblk1 : Inport
  cfblk15 : Inport  Port=2
  cfblk16 : Inport  Port=3
  cfblk10 : Subsystem
  cfblk11 : Subsystem
  cfblk12 : Subsystem
  cfblk13 : Subsystem
  cfblk14 : Subsystem
  cfblk18 : Delay  SampleTime=1
  cfblk19 : Delay  SampleTime=1
  cfblk20 : Delay  SampleTime=1
  cfblk3 : DiscreteFir  SampleTime=1
  cfblk4 : UnitDelay  HasFrameUpgradeWarning=on
  cfblk5 : DiscreteZeroPole  Poles=[0 0.5]  Gain=1
  cfblk6 : DiscreteFir  SampleTime=1
  cfblk7 : Sqrt  SaturateOnIntegerOverflow=on
  cfblk8 : Sum  Inputs=+
  cfblk9 : Constant  Value=[768188004.511148]  SampleTime=1
  cfblk2 : Outport
  cfblk17 : Outport  Port=2
  wires:
  cfblk15/1 -> cfblk13/1(cfblk1)
  cfblk8/1 -> cfblk5/1
  cfblk10/1(cfblk2) -> cfblk8/1
  cfblk3/1 -> cfblk4/1
  cfblk16/1 -> cfblk17/1
  cfblk9/1 -> cfblk3/1
  cfblk5/1 -> cfblk11/1(cfblk1)
  cfblk13/1(cfblk2) -> cfblk12/1(cfblk1)
  cfblk10/2(cfblk11) -> cfblk2/1
  cfblk14/1(cfblk2) -> cfblk12/2(cfblk17)
  cfblk7/1 -> cfblk10/2(cfblk10)
  cfblk14/2(cfblk8) -> cfblk6/1
  cfblk4/1 -> cfblk14/3(cfblk7)
  cfblk1/1 -> cfblk7/1
  cfblk11/1(cfblk2) -> cfblk18/1
  cfblk18/1 -> cfblk10/1(cfblk1)
  cfblk12/1(cfblk2) -> cfblk19/1
  cfblk19/1 -> cfblk14/1(cfblk1)
  cfblk6/1 -> cfblk20/1
  cfblk20/1 -> cfblk14/2(cfblk6)
